simulink model "model_no_bemf"  (R2015b)
settings: Solver=VariableStepAuto  StartTime=0.0  StopTime=10.0  RelTol=1e-3
InitFcn:
  | parameters
undefined symbols (not defined in the file): Ch, D, Ke, Kh, L, Mc, R
settings Model: Creator=gsavaia  LastModifiedBy=gsavaia

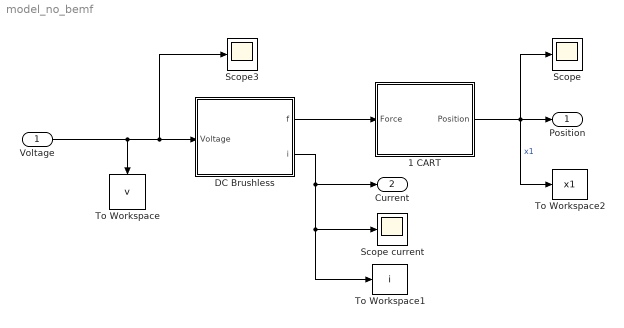
== system model_no_bemf ==
  "Voltage " : Inport
  1 CART : Subsystem
  DC Brushless : Subsystem
  Scope : Scope
  Scope current : Scope
  Scope3 : Scope
  To Workspace : ToWorkspace  VariableName=v  SaveFormat=Timeseries  SampleTime=-1
  To Workspace1 : ToWorkspace  VariableName=i  SaveFormat=Timeseries  SampleTime=-1
  To Workspace2 : ToWorkspace  VariableName=x1  SaveFormat=Timeseries  SampleTime=-1
  Position : Outport
  Current : Outport  Port=2
  wires:
  DC Brushless/1("f ") -> 1 CART/1(Force)
  1 CART/1(Position) -> Position/1, To Workspace2/1, Scope/1  "x1"
  "Voltage "/1 -> DC Brushless/1("Voltage "), Scope3/1, To Workspace/1
  DC Brushless/2(i) -> Current/1, To Workspace1/1, Scope current/1

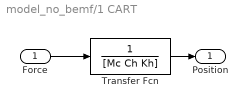
== system model_no_bemf/1 CART ==
  Force : Inport
  Transfer Fcn : TransferFcn  Denominator=[Mc Ch Kh]
  Position : Outport
  wires:
  Transfer Fcn/1 -> Position/1
  Force/1 -> Transfer Fcn/1

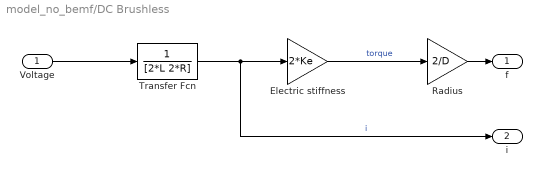
== system model_no_bemf/DC Brushless ==
  "Voltage " : Inport
  Electric stiffness : Gain  Gain=2*Ke
  Radius : Gain  Gain=2/D
  Transfer Fcn : TransferFcn  Denominator=[2*L 2*R]
  "f " : Outport
  i : Outport  Port=2
  wires:
  Transfer Fcn/1 -> i/1, Electric stiffness/1  "i"
  "Voltage "/1 -> Transfer Fcn/1
  Radius/1 -> "f "/1
  Electric stiffness/1 -> Radius/1  "torque"
